simulink model "PWM_Bridge"  (Simulink 7.5)
settings: Solver=ode45  StartTime=0.0  StopTime=0.01  RelTol=1e-3
libraries: powerlib x12, powerlib_extras x3, simulink x1
settings Model: Creator=lm  LastModifiedBy=lm

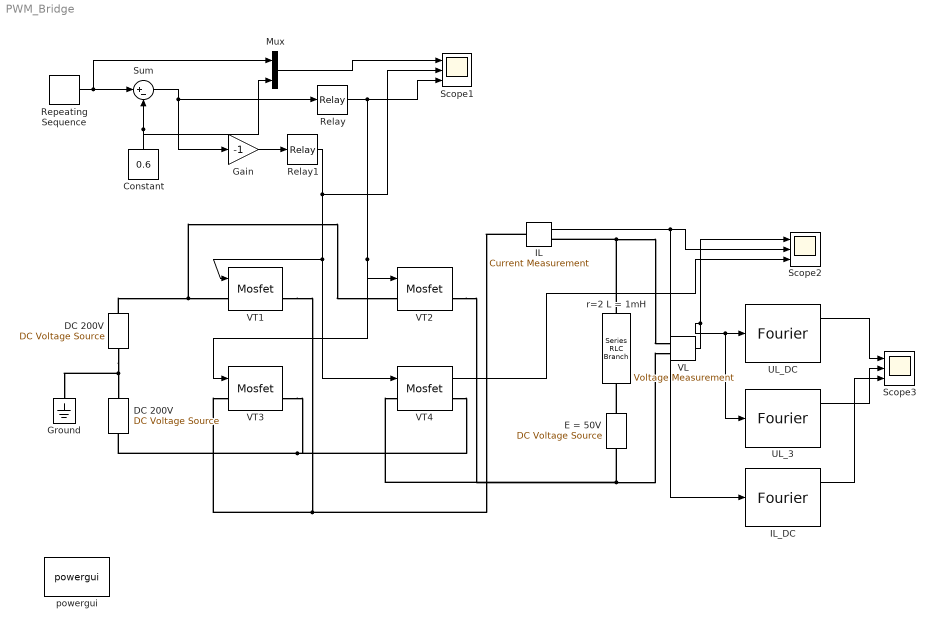
== system PWM_Bridge ==
  " DC 200V" : powerlib/Electrical Sources/DC Voltage Source  DialogController=POWERSYS.PowerSysDialog  SystemSampleTime=-1  Amplitude=200  Measurements=None
  Constant : Constant  Value=0.6  OutDataType=fixdt(1, 16)  OutScaling=2^0
  DC 200V : powerlib/Electrical Sources/DC Voltage Source  DialogController=POWERSYS.PowerSysDialog  SystemSampleTime=-1  Amplitude=200  Measurements=None
  E = 50V : powerlib/Electrical Sources/DC Voltage Source  DialogController=POWERSYS.PowerSysDialog  SystemSampleTime=-1  Amplitude=50  Measurements=None
  Gain : Gain  Gain=-1  ParameterDataType=fixdt(1, 16)  ParameterScaling=2^0  OutDataType=fixdt(1, 16)  OutScaling=2^0
  Ground : powerlib/Elements/Ground  DialogController=POWERSYS.PowerSysDialog  PhysicalDomain=powersysdomain  SubClassName=unknown  LeftPortType=p1  RightPortType=p1  LConnTagsString=a
  IL : powerlib/Measurements/Current Measurement  DialogController=POWERSYS.PowerSysDialog  SystemSampleTime=-1  PhasorSimulation=off  OutputType=Complex  PSBequivalent=0
  IL_DC : powerlib_extras/Measurements/Fourier  DialogController=POWERSYS.PowerSysDialog  SystemSampleTime=-1  f1=5000  n=0
  Mux : Mux  Inputs=2
  Relay : Relay  OnSwitchValue=1e-4  OffSwitchValue=-1e-4  OutDataType=fixdt(1, 16)  OutScaling=2^0
  Relay1 : Relay  OnSwitchValue=1e-4  OffSwitchValue=-1e-4  OutDataType=fixdt(1, 16)  OutScaling=2^0
  Repeating Sequence : simulink/Sources/Repeating Sequence  SystemSampleTime=-1  rep_seq_t=[0 1e-4]  rep_seq_y=[0 1]
  Scope1 : Scope  NumInputPorts=3
      settings: YMin=-2~-5~-5  YMax=2~5~5
  Scope2 : Scope  NumInputPorts=3
      settings: YMin=-5~0~-5  YMax=5~150~5  SaveName=ScopeData2
  Scope3 : Scope  NumInputPorts=3
      settings: YMin=-5~0~-5  YMax=5~150~5
  Sum : Sum  Inputs=|+-  OutDataType=fixdt(1, 16)  OutScaling=2^0
  UL_3 : powerlib_extras/Measurements/Fourier  DialogController=POWERSYS.PowerSysDialog  SystemSampleTime=-1  f1=5000  n=3
  UL_DC : powerlib_extras/Measurements/Fourier  DialogController=POWERSYS.PowerSysDialog  SystemSampleTime=-1  f1=5000  n=0
  VL : powerlib/Measurements/Voltage Measurement  DialogController=POWERSYS.PowerSysDialog  SystemSampleTime=-1  PhasorSimulation=off  OutputType=Complex  PSBequivalent=0
  VT{1..4} (4 alike) : powerlib/Power Electronics/Mosfet  DialogController=POWERSYS.PowerSysDialog  SystemSampleTime=-1  Ron=0.1  Lon=0  Rd=0.01  Vfd=0  IC=0  Rs=1e5  Cs=inf  Measurements=on
  powergui : powerlib/powergui  Priority=1  SystemSampleTime=-1  SimulationMode=Discrete  SampleTime=50e-6  frequency=60  SPID=off  DisableSnubberDevices=off  DisableRonSwitches=off  DisableVfSwitches=off  SwTol=0  Interpol=off  frequencyindice=0  echomessages=off  HookPort=off  DisplayEquations=off  FunctionMessages=off  EnableUseOfTLC=off  x0status=blocks  RestoreLinks=warning  ResistiveCurrentMeasurement=off  Ylog=off  Xlog=on  ShowGrid=off  save=off  variable=ZData  ZoomFFT=off  StartTime=0.0  cycles=1  DisplayStyle=1  FreqAxis=off  MaxFrequency=1000  frequencyindicesteady=1  display=off  methode=off
  r=2 L = 1mH : powerlib/Elements/Series RLC Branch  DialogController=POWERSYS.PowerSysDialog  PhysicalDomain=powersysdomain  SubClassName=unknown  LeftPortType=p1  RightPortType=p1  LConnTagsString=__new0  RConnTagsString=__new0  BranchType=RL  Resistance=2  Inductance=1e-3  SetiL0=off  InitialCurrent=0  Capacitance=1e-6  Setx0=off  InitialVoltage=0  Measurements=None
  wires:
  Repeating Sequence/1 -> Sum/1, Mux/1
  Constant/1 -> Sum/2, Mux/2
  Sum/1 -> Relay/1, Gain/1
  Gain/1 -> Relay1/1
  Relay1/1 -> VT1/1, VT4/1, Scope1/2
  Relay/1 -> VT2/1, VT3/1, Scope1/3
  VL/1 -> Scope2/1, UL_DC/1, UL_3/1
  IL/1 -> Scope2/2, IL_DC/1
  Mux/1 -> Scope1/1
  VT4/1 -> Scope2/3
  UL_DC/1 -> Scope3/1
  UL_3/1 -> Scope3/2
  IL_DC/1 -> Scope3/3
  connections:
  DC 200V/LConn1 -- " DC 200V"/RConn1 -- Ground/LConn1
  DC 200V/RConn1 -- VT1/LConn1 -- VT2/LConn1
  VT3/RConn1 -- " DC 200V"/LConn1 -- VT4/RConn1
  r=2 L = 1mH/LConn1 -- IL/RConn1 -- VL/LConn1
  IL/LConn1 -- VT3/LConn1 -- VT1/RConn1
  VT2/RConn1 -- VT4/LConn1 -- E = 50V/LConn1 -- VL/LConn2
  E = 50V/RConn1 -- r=2 L = 1mH/RConn1
